simulink model "model"  (R2023b)
settings: Solver=VariableStepAuto  StartTime=0.0  StopTime=100.0  RelTol=1e-3
values from neighbouring files (symbols this model uses):
  a = 0.01    [parametry.m]
  alfa = 0.5    [parametry.m]
  beta = 1    [parametry.m]
  K = 0.5    [parametry.m]
  k = 0.5    [parametry.m]
  m = 1    [parametry.m]
  w_0 = 0    [parametry.m]
  x_0 = 0.5    [parametry.m]
  x_prim_0 = 0    [parametry.m]
settings Model: Creator=student  LastModifiedBy=Jakub

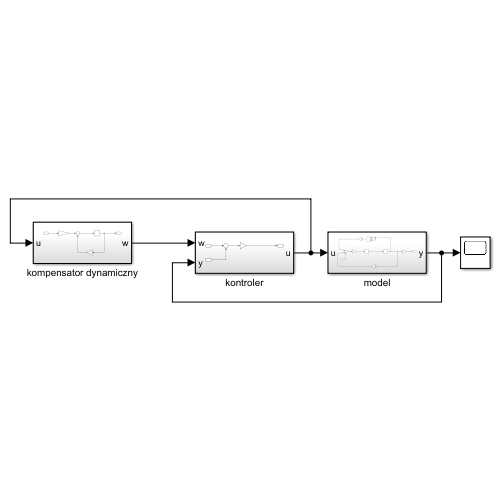
[thumbnail: Simulink's stored preview of the top-level diagram]
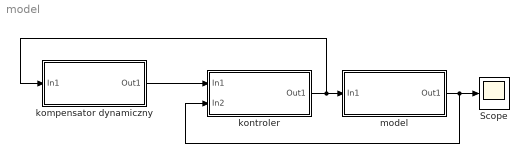
== system model ==
  Scope : Scope
  kompensator dynamiczny : Subsystem
  kontroler : Subsystem
  model : Subsystem
  wires:
  model/1(Out1) -> kontroler/2(In2), Scope/1
  kompensator dynamiczny/1(Out1) -> kontroler/1(In1)
  kontroler/1(Out1) -> kompensator dynamiczny/1(In1), model/1(In1)

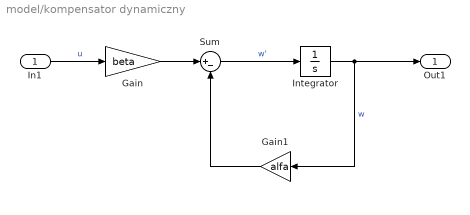
== system model/kompensator dynamiczny ==
  In1 : Inport
  Gain : Gain  Gain=beta
  Gain1 : Gain  Gain=alfa
  Integrator : Integrator  InitialCondition=w_0
  Sum : Sum  Inputs=|+-
  Out1 : Outport
  wires:
  In1/1 -> Gain/1  "u"
  Gain/1 -> Sum/1
  Integrator/1 -> Out1/1, Gain1/1  "w"
  Gain1/1 -> Sum/2
  Sum/1 -> Integrator/1  "w'"

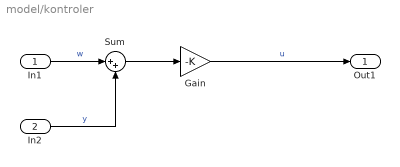
== system model/kontroler ==
  In1 : Inport
  In2 : Inport  Port=2
  Gain : Gain  Gain=-K
  Sum : Sum  Inputs=|++
  Out1 : Outport
  wires:
  Sum/1 -> Gain/1
  In1/1 -> Sum/1  "w"
  In2/1 -> Sum/2  "y"
  Gain/1 -> Out1/1  "u"

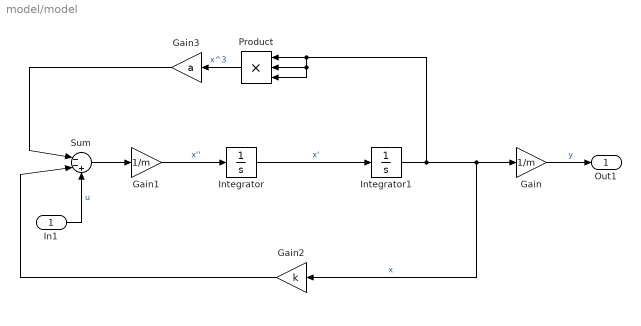
== system model/model ==
  In1 : Inport
  Gain : Gain  Gain=1/m
  Gain1 : Gain  Gain=1/m
  Gain2 : Gain  Gain=k
  Gain3 : Gain  Gain=a
  Integrator : Integrator  InitialCondition=x_prim_0
  Integrator1 : Integrator  InitialCondition=x_0
  Product : Product  Inputs=3
  Sum : Sum  Inputs=|--+
  Out1 : Outport
  wires:
  Gain1/1 -> Integrator/1  "x''"
  Integrator/1 -> Integrator1/1  "x'"
  Integrator1/1 -> Product/3, Product/2, Product/1, Gain2/1, Gain/1  "x"
  Gain/1 -> Out1/1  "y"
  Sum/1 -> Gain1/1
  Gain2/1 -> Sum/2
  Product/1 -> Gain3/1  "x^3"
  Gain3/1 -> Sum/1
  In1/1 -> Sum/3  "u"
